simulink model "simu1"  (R2020b)
settings: Solver=VariableStepAuto  StartTime=0.0  StopTime=15  MaxStep=0.01  RelTol=1e-3
values from neighbouring files (symbols this model uses):
  Kd = 2*xi*w*Jt    [Correction.m]
  Kp = Jt*w^2    (= 0.32934)    [Correction.m]
libraries: cstblocks x1
settings Model: Creator=d.alazard  LastModifiedBy=d.alazard

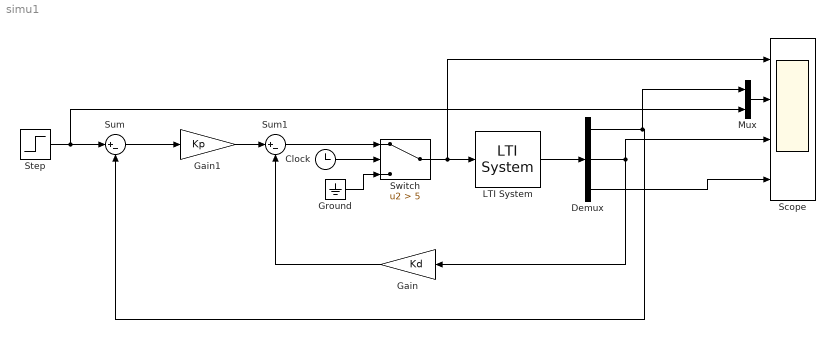
== system simu1 ==
  Clock : Clock
  Demux : Demux  Outputs=3
  Gain : Gain  Gain=Kd
  Gain1 : Gain  Gain=Kp
  Ground : Ground
  LTI System : cstblocks/LTI System  sys=sys  IC=x0
  Mux : Mux  Inputs=2
  Scope : Scope  NumInputPorts=4
  Step : Step  Time=10  After=10*pi/180  SampleTime=0
  Sum : Sum  Inputs=|+-
  Sum1 : Sum  Inputs=|+-
  Switch : Switch  Criteria=u2 > Threshold  Threshold=5
  wires:
  LTI System/1 -> Demux/1
  Gain1/1 -> Sum1/1
  Sum/1 -> Gain1/1
  Gain/1 -> Sum1/2
  Demux/2 -> Scope/3, Gain/1
  Demux/1 -> Mux/1, Sum/2
  Switch/1 -> Scope/1, LTI System/1
  Ground/1 -> Switch/3
  Clock/1 -> Switch/2
  Sum1/1 -> Switch/1
  Demux/3 -> Scope/4
  Mux/1 -> Scope/2
  Step/1 -> Mux/2, Sum/1
